simulink model "test"  (R2022b)
settings: Solver=VariableStepAuto  StartTime=0.0  StopTime=10  RelTol=1e-3
values from neighbouring files (symbols this model uses):
  A = [0 1 0 0; 0 0 m*g/M 0; 0 0 0 1; 0 0 (M+m)*g/(M*l) 0]    [invertpen_script_2.m]
  B = [0;1/M;0;1/l/M]    [invertpen_script_2.m]
  C = [1,0,0,0;0,0,1,0]    [invertpen_script_2.m]
  K = -1.0e+03 * [-0.0100    2.0280   -0.0641    0.0591]    [invertpen_script.m]    (also in invertpen_script_2.m = -1*lqr(A,B,Q,R))
  L = -1*FO_observer    [invertpen_script_2.m]
settings Model: Creator=lizehua2  LastModifiedBy=kevin
settings SolverCC: AlgebraicLoopSolver=TrustRegion
settings DataIOCC: ReturnWorkspaceOutputs=off
settings DebuggingCC: UnconnectedInputMsg=warning  UnconnectedOutputMsg=warning  UnconnectedLineMsg=warning  SFMachineParentedDataDiag=warning  ArithmeticOperatorsInVariantConditions=warning
settings ModelReferenceCC: EnableRefExpFcnMdlSchedulingChecks=on
settings SFSimCC: SimUseLocalCustomCode=off  CustomCodeUndefinedFunction=UseInterfaceOnly
settings RTWCC: RTWUseLocalCustomCode=off

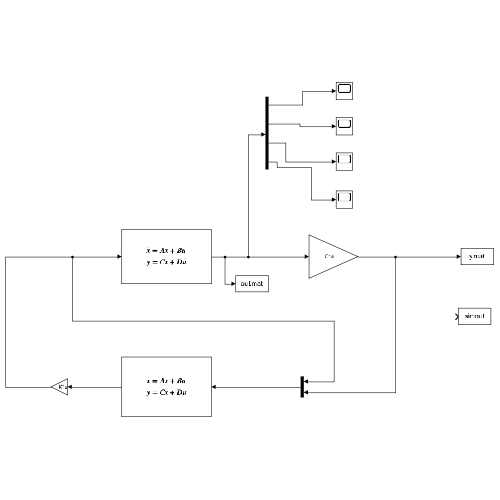
[thumbnail: Simulink's stored preview of the top-level diagram]
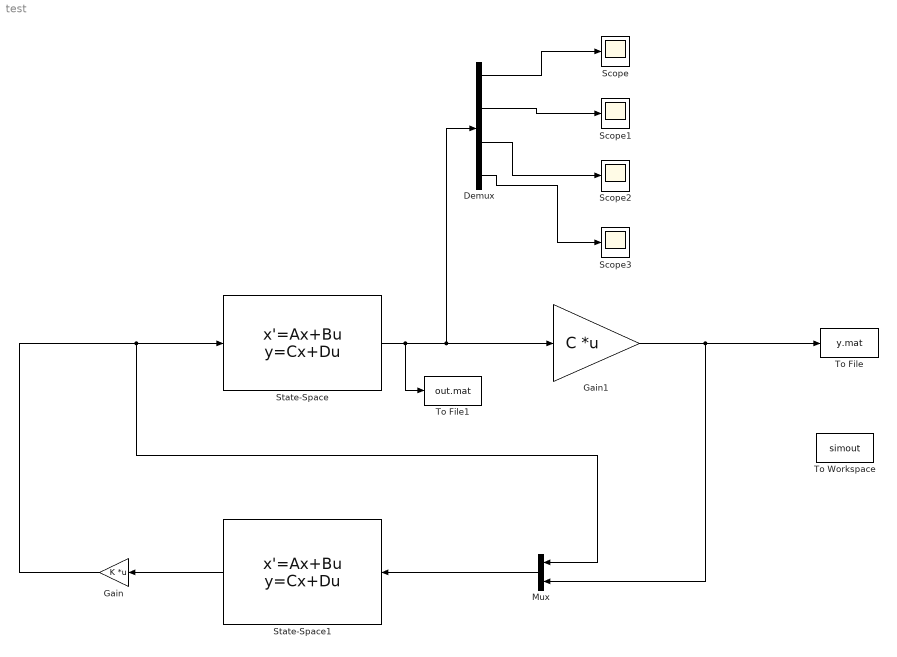
== system test ==
  Demux : Demux
  Gain : Gain  Gain=K  Multiplication=Matrix(K*u)
  Gain1 : Gain  Gain=C  Multiplication=Matrix(K*u)
  Mux : Mux  Inputs=2
  Scope{,1..3} (4 alike) : Scope
  State-Space : StateSpace  A=A  B=B  C=eye(4)  D=zeros(4,1)  InitialCondition=[0.5;0.1;0.175;0]
  State-Space1 : StateSpace  A=A-L*C  B=[B L]  C=eye(4)  D=zeros(4,3)  InitialCondition=[0.5;0.1;0.175;0]
  To File : ToFile  Filename=y.mat  MatrixName=y  SaveFormat=Timeseries
  To File1 : ToFile  Filename=out.mat  MatrixName=output
  To Workspace : ToWorkspace  VariableName=simout  SaveFormat=Timeseries  SampleTime=-1
  wires:
  State-Space1/1 -> Gain/1
  Gain/1 -> State-Space/1, Mux/1
  State-Space/1 -> To File1/1, Demux/1, Gain1/1
  Gain1/1 -> Mux/2, To File/1
  Mux/1 -> State-Space1/1
  Demux/1 -> Scope/1
  Demux/2 -> Scope1/1
  Demux/3 -> Scope2/1
  Demux/4 -> Scope3/1
